simulink model "tanque_PID"  (R2017a)
settings: Solver=ode45  StartTime=0.0  StopTime=1000  RelTol=1e-3  EnableMultiTasking=on
values from neighbouring files (symbols this model uses):
  k1 = k_bar*inv(Co)*phi    [Realimentacion_Acker.m]
  k2 = acker(A,b,Ed)    [Realimentacion_Acker.m]
  Kc = 0.6*Ku/type    [PID_Ku.m]
  N = [C;C*A;C*A^2]    [Smulacro_Parcial_Final.m]
  td = Tu/8    [PID_Ku.m]
  ti = Tu/2    [PID_Ku.m]
undefined symbols (not defined in the file or in its folder): A1, A2, a2s, h1s, h2s, k3
libraries: simulink x2
settings Model: Creator=Sergio  LastModifiedBy=Sergio
settings DataIOCC: LimitDataPoints=on  SaveFormat=Array  SignalLoggingSaveFormat=ModelDataLogs
settings OptimizationCC: ExpressionDepthLimit=2147483647  LifeSpan=inf
settings DebuggingCC: UnderspecifiedInitializationDetection=Classic  MergeDetectMultiDrivingBlocksExec=none  SolverPrmCheckMsg=warning  FcnCallInpInsideContextMsg=warning  StateNameClashWarn=warning  SFUnexpectedBacktrackingDiag=warning  SFNoUnconditionalDefaultTransitionDiag=warning  SFExecutionAtInitializationDiag=none
settings HardwareCC: ProdBitPerPointer=32  ProdBitPerSizeT=32  ProdBitPerPtrDiffT=32  ProdLargestAtomicFloat=None  ProdIntDivRoundTo=Undefined  ProdEndianess=Unspecified  ProdWordSize=32  ProdHWDeviceType=32-bit Generic
settings ModelReferenceCC: PropagateSignalLabelsOutOfModel=off
settings GRTTargetCC: TargetLangStandard=C89/C90 (ANSI)  GeneratePreprocessorConditionals=Disable all
settings ConfigComp: CovMetricSettings=dw  CovHtmlReporting=on  CovSaveCumulativeToWorkspaceVar=on  CovSaveSingleToWorkspaceVar=on  CovExternalEMLEnable=off  CovSFcnEnable=off

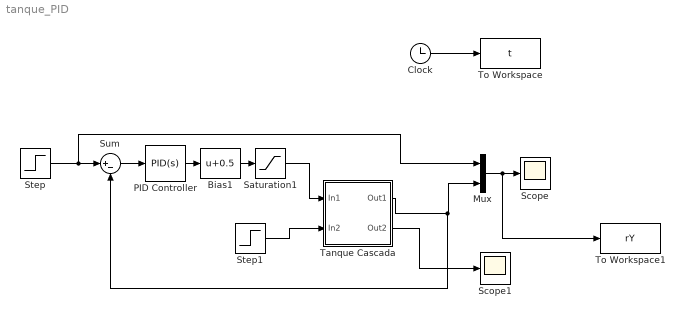
== system tanque_PID ==
  Bias1 : Bias  Bias=0.5
  Clock : Clock
  Mux : Mux  Inputs=2
  PID Controller : simulink/Continuous/PID Controller  Controller=PID  TimeDomain=Continuous-time  SampleTime=-1  IntegratorMethod=Forward Euler  FilterMethod=Forward Euler  Form=Ideal  UseFilter=on  ControllerParametersSource=internal  P=Kc  I=1/ti  D=td  N=N  InitialConditionSource=internal  InitialConditionForIntegrator=0  InitialConditionForFilter=0  ExternalReset=none  LimitOutput=off  UpperSaturationLimit=inf  LowerSaturationLimit=-inf  LinearizeAsGain=on  AntiWindupMode=none  Kb=1  TrackingMode=off  Kt=1  PParamMin=[]  PParamMax=[]  IParamMin=[]  IParamMax=[]  DParamMin=[]  DParamMax=[]  NParamMin=[]  NParamMax=[]  KbParamMin=[]  KbParamMax=[]  KtParamMin=[]  KtParamMax=[]  POutMin=[]  POutMax=[]  IOutMin=[]  IOutMax=[]  DOutMin=[]  DOutMax=[]  NOutMin=[]  NOutMax=[]  KbOutMin=[]  KbOutMax=[]  KtOutMin=[]  KtOutMax=[]  IntegratorOutMin=[]  IntegratorOutMax=[]  FilterOutMin=[]  FilterOutMax=[]  SumOutMin=[]  SumOutMax=[]  SumI1OutMin=[]  SumI1OutMax=[]  SumI2OutMin=[]  SumI2OutMax=[]  SumI3OutMin=[]  SumI3OutMax=[]  SumDOutMin=[]  SumDOutMax=[]  SaturationOutMin=[]  SaturationOutMax=[]  IntegratorContinuousStateAttributes=''  IntegratorStateMustResolveToSignalObject=off  IntegratorRTWStateStorageClass=Auto  FilterContinuousStateAttributes=''  FilterStateMustResolveToSignalObject=off  FilterRTWStateStorageClass=Auto  DifferentiatorICPrevScaledInput=0  DifferentiatorOutMin=[]  DifferentiatorOutMax=[]  InitialConditionSetting=State (most efficient)
  Saturation1 : Saturate  UpperLimit=1  LowerLimit=0
  Scope : Scope
  Scope1 : Scope
  Step : Step  Time=50  Before=0.653  After=0.7  SampleTime=0
  Step1 : Step  Time=600  Before=a2s  After=a2s-0.02  SampleTime=0
  Sum : Sum  Inputs=|+-
  Tanque Cascada : Subsystem
  To Workspace : ToWorkspace  VariableName=t  SampleTime=-1
  To Workspace1 : ToWorkspace  VariableName=rY  SampleTime=-1
  wires:
  Clock/1 -> To Workspace/1
  Step1/1 -> Tanque Cascada/2(In2)
  Sum/1 -> PID Controller/1
  Tanque Cascada/1(Out1) -> Sum/2, Mux/2
  Mux/1 -> To Workspace1/1, Scope/1
  Step/1 -> Sum/1, Mux/1
  PID Controller/1 -> Bias1/1
  Bias1/1 -> Saturation1/1
  Saturation1/1 -> Tanque Cascada/1(In1)
  Tanque Cascada/2(Out2) -> Scope1/1

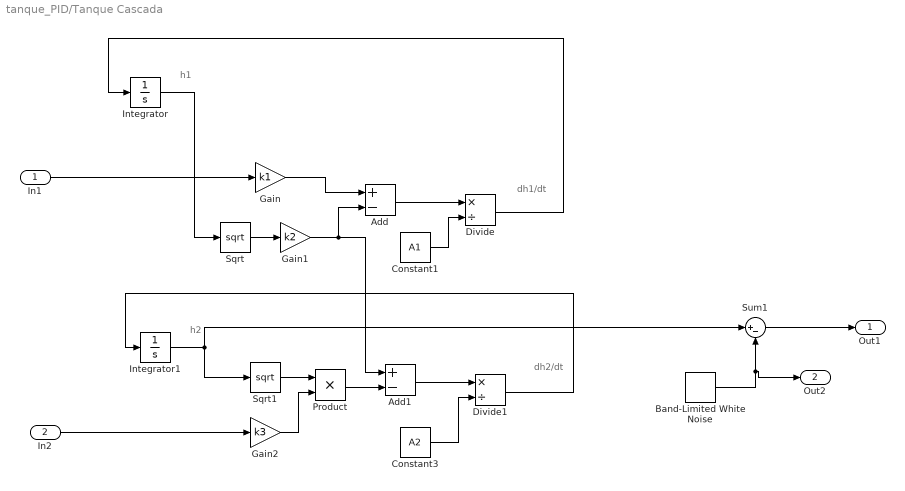
== system tanque_PID/Tanque Cascada ==
  note: dh1/dt
  note: h1
  note: dh2/dt
  note: h2
  In1 : Inport
  In2 : Inport  Port=2
  Add : Sum  Inputs=+-
  Add1 : Sum  Inputs=+-
  Band-Limited White Noise : simulink/Sources/Band-Limited White Noise  Cov=[0.0000001]  Ts=0.1  seed=[23341]
  Constant1 : Constant  Value=A1
  Constant3 : Constant  Value=A2
  Divide : Product  Inputs=*/
  Divide1 : Product  Inputs=*/
  Gain : Gain  Gain=k1
  Gain1 : Gain  Gain=k2
  Gain2 : Gain  Gain=k3
  Integrator : Integrator  InitialCondition=h1s
  Integrator1 : Integrator  InitialCondition=h2s
  Product : Product
  Sqrt : Sqrt  SaturateOnIntegerOverflow=on
  Sqrt1 : Sqrt  SaturateOnIntegerOverflow=on
  Sum1 : Sum  Inputs=|+-
  Out1 : Outport
  Out2 : Outport  Port=2
  wires:
  Integrator/1 -> Sqrt/1
  In1/1 -> Gain/1
  Gain2/1 -> Product/2
  Add/1 -> Divide/1
  Product/1 -> Add1/2
  Gain1/1 -> Add1/1, Add/2
  Divide/1 -> Integrator/1
  Constant1/1 -> Divide/2
  Gain/1 -> Add/1
  Sqrt/1 -> Gain1/1
  Add1/1 -> Divide1/1
  Sqrt1/1 -> Product/1
  Constant3/1 -> Divide1/2
  In2/1 -> Gain2/1
  Divide1/1 -> Integrator1/1
  Band-Limited White Noise/1 -> Out2/1, Sum1/2
  Sum1/1 -> Out1/1
  Integrator1/1 -> Sqrt1/1, Sum1/1
